simulink model "AutoEncoderPredictSim"  (R2022a)
settings: Solver=VariableStepAuto  StartTime=0.0  StopTime=labels.Length  RelTol=1e-3
undefined symbols (not defined in the file or in its folder): threshold
libraries: simulink x1, matrix_library x1, dspstat3 x1, deeplib x1
settings Model: Creator=Alia  LastModifiedBy=adria
settings SolverCC: AlgebraicLoopSolver=TrustRegion
settings DebuggingCC: UnconnectedInputMsg=warning  UnconnectedOutputMsg=warning  UnconnectedLineMsg=warning  SFMachineParentedDataDiag=warning
settings RTWCC: DLArmComputeVersion=19.05

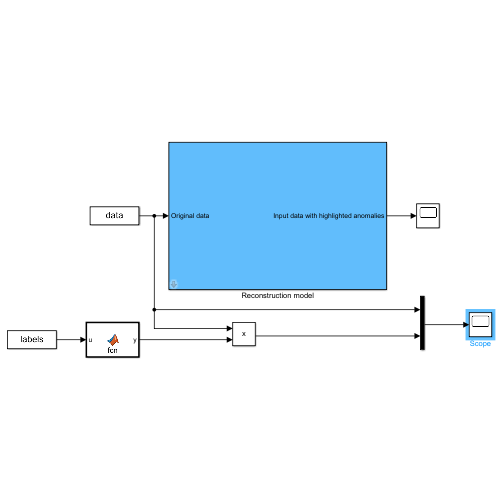
[thumbnail: Simulink's stored preview of the top-level diagram]
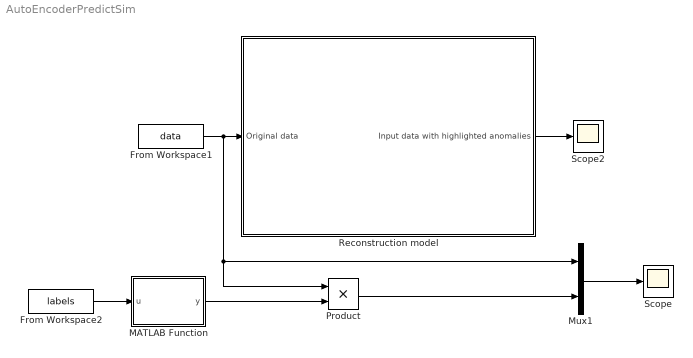
== system AutoEncoderPredictSim ==
  From Workspace1 : FromWorkspace  VariableName=data
  From Workspace2 : FromWorkspace  VariableName=labels
  MATLAB Function : MATLAB Function  TreatAsAtomicUnit=on
  Mux1 : Mux  Inputs=2
  Product : Product
  Reconstruction model : Subsystem  mask{BufferLength=35, NetworkFilePath=D:\Personen\Ich\Studium\Bachelorarbeit\Inhalt\Git\Output\net.mat, InputDataFormats={ '', '' }}
      mask prompts: BufferLength "dspshared:blkprm_prompts:OutputBufferSize"; NetworkFilePath "deep_blocks:common:FilePath"; InputDataFormats "deep_blocks:predict:InputDataFormats"
      mask help: Buffer overload value must be equal to 1-BufferSize
      mask TypeOptions BufferLength:
      | Buffer timestamps/Buffer/N | Delay/DelayLength | Compare values to theshold/Compare
      | To Constant/const
      mask TypeOptions NetworkFilePath: Reconstruction network/NetworkFilePath | Reconstruction network/NetworkFunction
      mask TypeOptions InputDataFormats: Reconstruction network/InputDataFormats
      mask DialogControl BufferLength Prompt: Output buffer size (per channel):
      mask DialogControl NetworkFilePath Prompt: File path:
      mask DialogControl Control2 Prompt: Browse
      mask DialogControl InputDataFormats Prompt: Input data formats:
  Scope : Scope
  Scope2 : Scope
  wires:
  Mux1/1 -> Scope/1
  MATLAB Function/1(y) -> Product/2
  Reconstruction model/1(Input data with highlighted anomalies) -> Scope2/1
  Product/1 -> Mux1/2
  From Workspace2/1 -> MATLAB Function/1(u)
  From Workspace1/1 -> Mux1/1, Product/1, Reconstruction model/1(Original data)

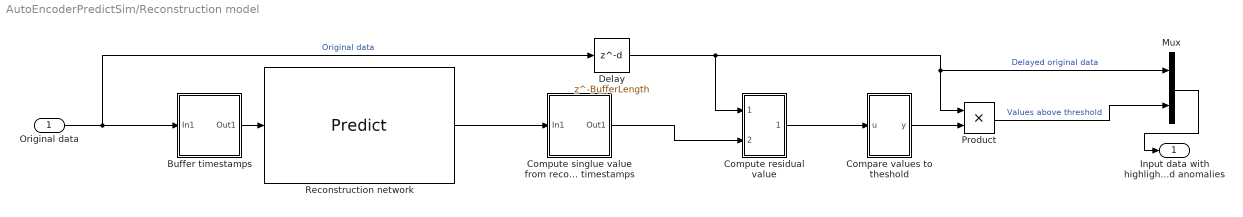
== system AutoEncoderPredictSim/Reconstruction model ==
  Original data : Inport
  Buffer timestamps : Subsystem
  Compare values to theshold : Subsystem
  Compute residual value : Subsystem
  Compute singlue value from reconstructed timestamps : Subsystem
  Delay : Delay  DelayLength=BufferLength
  Mux : Mux  Inputs=2
  Product : Product
  Reconstruction network : deeplib/Predict  Network=Network from MAT-file  NetworkFunction=D:\Personen\Ich\Studium\Bachelorarbeit\Inhalt\Git\Output\net.mat  NetworkFilePath=D:\Personen\Ich\Studium\Bachelorarbeit\Inhalt\Git\Output\net.mat  MiniBatchSize=128  InputDataFormats={ '', '' }  Predictions=on  Activations={}  ForceInterpretedSim=off  EnableDLNetwork=off
      settings: SourceProductBaseCode=NN
  Input data with highlighted anomalies : Outport
  wires:
  Compare values to theshold/1(y) -> Product/2
  Buffer timestamps/1(Out1) -> Reconstruction network/1
  Compute residual value/1(Out1) -> Compare values to theshold/1(u)
  Original data/1 -> Delay/1, Buffer timestamps/1(In1)  "Original data"
  Compute singlue value from reconstructed timestamps/1(Out1) -> Compute residual value/2(In2)
  Delay/1 -> Product/1, Mux/1, Compute residual value/1(In1)  "Delayed original data"
  Reconstruction network/1 -> Compute singlue value from reconstructed timestamps/1(In1)
  Mux/1 -> Input data with highlighted anomalies/1
  Product/1 -> Mux/2  "Values above threshold"

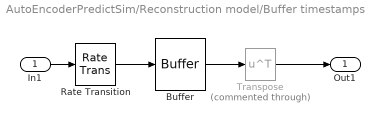
== system AutoEncoderPredictSim/Reconstruction model/Buffer timestamps ==
  In1 : Inport
  Buffer : Buffer  N=BufferLength  V=BufferLength-1  OutputFrames=off
  Rate Transition : RateTransition  OutPortSampleTime=1
  Transpose : Math  Commented=through  Operator=transpose
  Out1 : Outport
  wires:
  Rate Transition/1 -> Buffer/1
  Buffer/1 -> Transpose/1
  In1/1 -> Rate Transition/1
  Transpose/1 -> Out1/1

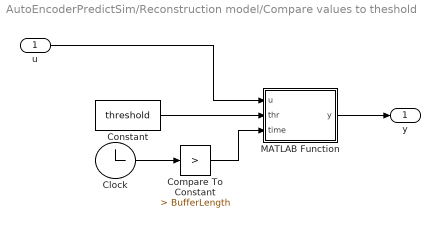
== system AutoEncoderPredictSim/Reconstruction model/Compare values to theshold ==
  u : Inport
  Clock : Clock
  Compare To Constant : simulink/Logic and Bit Operations/Compare To Constant  relop=>  const=BufferLength  OutDataTypeStr=boolean
  Constant : Constant  Value=threshold
  MATLAB Function : MATLAB Function  TreatAsAtomicUnit=on
  y : Outport
  wires:
  Clock/1 -> Compare To Constant/1
  Compare To Constant/1 -> MATLAB Function/3(time)
  Constant/1 -> MATLAB Function/2(thr)
  u/1 -> MATLAB Function/1(u)
  MATLAB Function/1(y) -> y/1

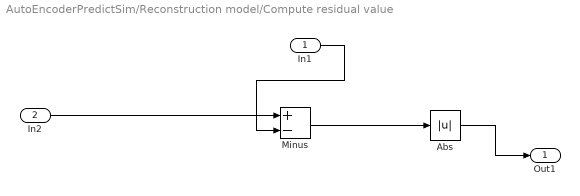
== system AutoEncoderPredictSim/Reconstruction model/Compute residual value ==
  In1 : Inport
  In2 : Inport  Port=2
  Abs : Abs  SaturateOnIntegerOverflow=off
  Minus : Sum  Inputs=+-
  Out1 : Outport
  wires:
  In1/1 -> Minus/2
  Minus/1 -> Abs/1
  In2/1 -> Minus/1
  Abs/1 -> Out1/1

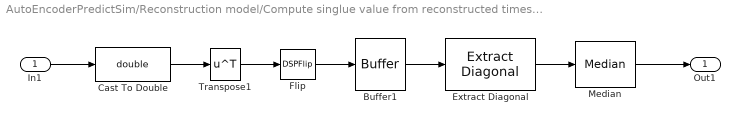
== system AutoEncoderPredictSim/Reconstruction model/Compute singlue value from reconstructed timestamps ==
  In1 : Inport
  Buffer1 : Buffer  N=BufferLength  V=BufferLength-1  OutputFrames=off
  Cast To Double : DataTypeConversion  OutDataTypeStr=double  SaturateOnIntegerOverflow=off  RndMeth=Floor
  Extract Diagonal : matrix_library/Extract Diagonal
      settings: SourceProductBaseCode=SL
  Flip : DSPFlip
  Median : dspstat3/Median  sortAlg=Quick sort  directionMode=Each column  dimension=1  roundingMode=Floor  overflowMode=off  accumDataTypeStr=Inherit: Same as product output  accumLastDataTypeStr=Inherit: Same as product output  outputDataTypeStr=Inherit: Same as accumulator  outputMin=[]  outputMax=[]  outputLastDataTypeStr=Inherit: Same as accumulator
      settings: SourceProductBaseCode=DS  allowOverrides=off
  Transpose1 : Math  Operator=transpose
  Out1 : Outport
  wires:
  Flip/1 -> Buffer1/1
  Buffer1/1 -> Extract Diagonal/1
  Transpose1/1 -> Flip/1
  In1/1 -> Cast To Double/1
  Extract Diagonal/1 -> Median/1
  Cast To Double/1 -> Transpose1/1
  Median/1 -> Out1/1

== matlab function AutoEncoderPredictSim/MATLAB Function ==
  data: u input; y output
function y = fcn(u)
y = NaN;
if u == 1
    y = 1;
end

== matlab function AutoEncoderPredictSim/Reconstruction model/Compare values to theshold/MATLAB Function ==
  data: u input; y output; thr input; time input
function y = fcn(u,thr, time)
y = NaN;
if time == 1
    if u > thr
    y = 1;
    end
end
